simulink model "Project_SADC"  (R2021b)
settings: Solver=ode45  StartTime=0.0  StopTime=T  FixedStep=1e-6  RelTol=1e-12
values from neighbouring files (symbols this model uses):
  A = [A_sc,A_sp]    [Main_SADC_10572571.m]
  Abn0 = Anb0'    [Main_SADC_10572571.m]
  epsilon = deg2rad(23.45)    [Main_SADC_10572571.m]
  m = [0.01 0.05 0.01]'    [Main_SADC_10572571.m]
  N = [n1 n2 n3 n4 n5 n6 n7 n8 n9 n10]    [Main_SADC_10572571.m]
  n_sun = 2*pi / T_sun    (= 1.99238499086e-07)    [Main_SADC_10572571.m]
  P_srp = Fe_tot/c    [Main_SADC_10572571.m]
  R3H0 = data.Re^3*H0    [Main_SADC_10572571.m]
  R_sun = astroConstants(2)    [Main_SADC_10572571.m]
  rho_d = cat(2,ones(1,6)*rho_d_sc,ones(1,4)*rho_d_sp)    [Main_SADC_10572571.m]
  rho_s = cat(2,ones(1,6)*rho_s_sc,ones(1,4)*rho_s_sp)    [Main_SADC_10572571.m]
  ri = [ri_sc,r_sp1,r_sp1,r_sp2,r_sp2]    [Main_SADC_10572571.m]
  w0 = [wx0 wy0 wz0]'    [Main_SADC_10572571.m]
  weights = [0.15;0.5;0.35]    [Main_SADC_10572571.m]
undefined symbols (not defined in the file or in its folder): data, gyro, horizonsensor, magnetometer, rr0, sc, sunsensor, vv0, wheel
libraries: simulink_extras x10
(part 2 of 3)

== system Project_SADC/Attitude determination /selection sensor/If Action Subsystem3 ==
  In1 : Inport
  Action Port : ActionPort
  Out1 : Outport
  wires:
  In1/1 -> Out1/1

== system Project_SADC/Attitude determination /selection sensor/Vector norm3 ==
  u : Inport
  Divide : Product  Inputs=*/
  norm_vector : Subsystem
  u_versor : Outport
  ||u|| : Outport  Port=2
  wires:
  Divide/1 -> u_versor/1
  norm_vector/1(|u|) -> Divide/2, ||u||/1
  u/1 -> norm_vector/1(u), Divide/1

== system Project_SADC/Euler equations/product vector/i-component ==
  A : Inport
  B : Inport  Port=2
  Demux : Demux  Outputs=3
  Demux1 : Demux  Outputs=3
  Product : Product
  Product1 : Product
  Sum : Sum  Inputs=+-
  Terminator : Terminator
  Terminator1 : Terminator
  Out2 : Outport
  wires:
  Sum/1 -> Out2/1
  Product1/1 -> Sum/2  "a3b2"
  Demux1/2 -> Product1/2  "b2"
  Product/1 -> Sum/1  "a2b3"
  Demux/2 -> Product/1  "a2"
  Demux/3 -> Product1/1  "a3"
  Demux1/3 -> Product/2  "b3"
  Demux/1 -> Terminator/1  "a1"
  Demux1/1 -> Terminator1/1
  B/1 -> Demux1/1
  A/1 -> Demux/1

== system Project_SADC/Euler equations/product vector/j-component ==
  A : Inport
  B : Inport  Port=2
  Demux : Demux  Outputs=3
  Demux1 : Demux  Outputs=3
  Product : Product
  Product1 : Product
  Sum : Sum  Inputs=+-
  Terminator : Terminator
  Terminator1 : Terminator
  Out1 : Outport
  wires:
  B/1 -> Demux1/1
  A/1 -> Demux/1
  Demux/3 -> Product/1  "a3"
  Demux1/1 -> Product/2  "b1"
  Demux/1 -> Product1/1  "a1"
  Demux1/3 -> Product1/2  "b3"
  Demux1/2 -> Terminator/1
  Demux/2 -> Terminator1/1
  Product/1 -> Sum/1
  Product1/1 -> Sum/2
  Sum/1 -> Out1/1

== system Project_SADC/Euler equations/product vector/k-component1 ==
  A : Inport
  B : Inport  Port=2
  Demux : Demux  Outputs=3
  Demux1 : Demux  Outputs=3
  Product : Product
  Product1 : Product
  Sum : Sum  Inputs=+-
  Terminator : Terminator
  Terminator1 : Terminator
  Out1 : Outport
  wires:
  Sum/1 -> Out1/1
  Product1/1 -> Sum/2
  Product/1 -> Sum/1
  Demux1/2 -> Product/2  "b2"
  A/1 -> Demux/1
  B/1 -> Demux1/1
  Demux/1 -> Product/1  "a1"
  Demux/2 -> Product1/1  "a2"
  Demux1/1 -> Product1/2  "b1"
  Demux1/3 -> Terminator/1  "b3"
  Demux/3 -> Terminator1/1  "a3"

== system Project_SADC/External torques/GG torque/Vector norm ==
  u : Inport
  Divide : Product  Inputs=*/
  norm_vector : Subsystem
  u_versor : Outport
  ||u|| : Outport  Port=2
  wires:
  u/1 -> Divide/1, norm_vector/1(u)
  norm_vector/1(|u|) -> ||u||/1, Divide/2
  Divide/1 -> u_versor/1

== system Project_SADC/External torques/GG torque/product vector ==
  A : Inport
  B : Inport  Port=2
  Mux : Mux  Inputs=3
  i-component : Subsystem
  j-component : Subsystem
  k-component1 : Subsystem
  C : Outport
  wires:
  Mux/1 -> C/1
  A/1 -> k-component1/1(A), j-component/1(A), i-component/1(A)
  B/1 -> k-component1/2(B), j-component/2(B), i-component/2(B)
  i-component/1(Out2) -> Mux/1
  j-component/1(Out1) -> Mux/2
  k-component1/1(Out1) -> Mux/3

== system Project_SADC/External torques/Magnetic torque/mag_field in inertial ==
  r_vect : Inport
  time : Inport  Port=2
  Constant : Constant  Value=3
  Constant1 : Constant  Value=R3H0
  Dot Product : DotProduct  InputSameDT=on  OutDataTypeStr=Inherit: Inherit via internal rule
  Gain : Gain  Gain=3
  MatrixMultiply : Product
  MatrixMultiply1 : Product
  Power : Math  Operator=pow  SaturateOnIntegerOverflow=on
  Product : Product  Inputs=/*
  Sum : Sum  Inputs=+-
  Vector norm1 : Subsystem
  m_versor : Subsystem
  b_B : Outport
  wires:
  r_vect/1 -> Vector norm1/1(u)
  time/1 -> m_versor/1(time)
  Vector norm1/2(||u||) -> Power/1
  Constant/1 -> Power/2
  Power/1 -> Product/1
  Constant1/1 -> Product/2
  m_versor/1(m) -> Sum/2, Dot Product/1
  Vector norm1/1(u_versor) -> MatrixMultiply/2, Dot Product/2
  MatrixMultiply/1 -> Sum/1
  Sum/1 -> MatrixMultiply1/1
  Product/1 -> MatrixMultiply1/2
  MatrixMultiply1/1 -> b_B/1
  Dot Product/1 -> Gain/1
  Gain/1 -> MatrixMultiply/1

== system Project_SADC/External torques/Magnetic torque/product vector2 ==
  A : Inport
  B : Inport  Port=2
  Mux : Mux  Inputs=3
  i-component : Subsystem
  j-component : Subsystem
  k-component1 : Subsystem
  C : Outport
  wires:
  k-component1/1(Out1) -> Mux/3
  j-component/1(Out1) -> Mux/2
  i-component/1(Out2) -> Mux/1
  B/1 -> i-component/2(B), j-component/2(B), k-component1/2(B)
  A/1 -> i-component/1(A), j-component/1(A), k-component1/1(A)
  Mux/1 -> C/1

== system Project_SADC/External torques/SRP torque/SRP forces ==
  r_Sun : Inport
  Constant : Constant  Value=1-rho_s  VectorParams1D=off
  Constant1 : Constant  Value=2.*rho_s  VectorParams1D=off
  Constant2 : Constant  Value=N  VectorParams1D=off
  Constant3 : Constant  Value=rho_d.*2./3  VectorParams1D=off
  Constant4 : Constant  Value=ones(1,10)  VectorParams1D=off
  Constant5 : Constant  Value=A  VectorParams1D=off
  Display : Display
  Element-wise([1x9].*[3x9])1 : Subsystem
  Element-wise([1x9].*[3x9])2 : Subsystem
  Element-wise([1x9].*[3x9])3 : Subsystem
  Gain : Gain  Gain=-P_srp
  MatrixMultiply : Product
  MatrixMultiply1 : Product  Multiplication=Matrix(*)
  MatrixMultiply2 : Product
  Subsystem : Subsystem
  Sum : Sum
  Sum1 : Sum
  Terminator : Terminator
  Vector norm1 : Subsystem
  F_srp : Outport
  S_dot_N : Outport  Port=2
  wires:
  Subsystem/1(S_dot_N) -> MatrixMultiply2/1, S_dot_N/1, MatrixMultiply/2
  Constant1/1 -> MatrixMultiply/1
  MatrixMultiply/1 -> Sum/2
  Constant3/1 -> Sum/1
  Constant2/1 -> Element-wise([1x9].*[3x9])3/1(N), Subsystem/2(N)
  Sum/1 -> Element-wise([1x9].*[3x9])3/2(vector)
  Constant4/1 -> MatrixMultiply1/2
  MatrixMultiply1/1 -> Element-wise([1x9].*[3x9])1/1(Sb)
  Constant/1 -> Display/1, Element-wise([1x9].*[3x9])1/2(vector)
  Element-wise([1x9].*[3x9])1/1(vect.*Sb) -> Sum1/1
  Element-wise([1x9].*[3x9])3/1(vect.*n) -> Sum1/2
  Constant5/1 -> Gain/1
  Gain/1 -> MatrixMultiply2/2
  Sum1/1 -> Element-wise([1x9].*[3x9])2/1(mat)
  MatrixMultiply2/1 -> Element-wise([1x9].*[3x9])2/2(vector)
  Element-wise([1x9].*[3x9])2/1(vect.*mat) -> F_srp/1
  r_Sun/1 -> Vector norm1/1(u)
  Vector norm1/1(u_versor) -> MatrixMultiply1/1, Subsystem/1(r_sun)
  Vector norm1/2(||u||) -> Terminator/1

== system Project_SADC/External torques/SRP torque/Sun wrt s//c ==
  A_BN : Inport
  r_vect : Inport  Port=2
  t : Inport  Port=3
  MatrixMultiply : Product  Multiplication=Matrix(*)
  R_Sun in inertial : Subsystem
  Sum : Sum  Inputs=-+
  To Workspace : ToWorkspace  VariableName=r_Sun_N  SaveFormat=Timeseries  SampleTime=-1
  r_sun : Outport
  rSun_N : Outport  Port=2
  wires:
  t/1 -> R_Sun in inertial/1(t)
  r_vect/1 -> Sum/1
  R_Sun in inertial/1(R_sun_N) -> rSun_N/1, To Workspace/1, Sum/2
  Sum/1 -> MatrixMultiply/2
  A_BN/1 -> MatrixMultiply/1
  MatrixMultiply/1 -> r_sun/1  "R_Sun in body"

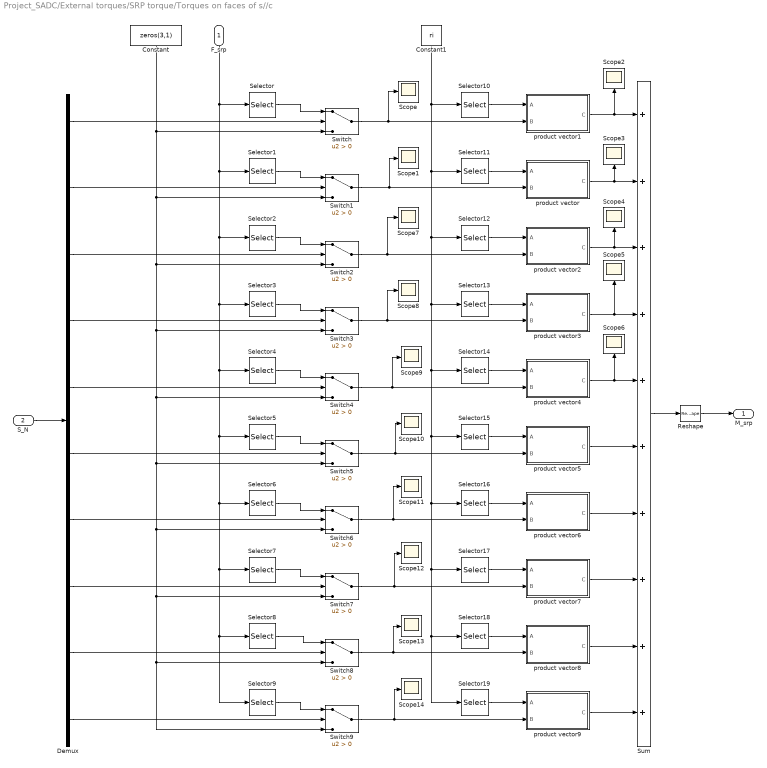
== system Project_SADC/External torques/SRP torque/Torques on faces of s//c ==
  F_srp : Inport
  S_N : Inport  Port=2
  Constant : Constant  Value=zeros(3,1)
  Constant1 : Constant  Value=ri
  Demux : Demux  Outputs=10
  Reshape : Reshape  OutputDimensionality=Column vector (2-D)
  Scope{,1..14} (15 alike) : Scope
  Selector : Selector  NumberOfDimensions=2  InputPortWidth=3  IndexOptions=Index vector (dialog),Index vector (dialog)  Indices=[1 2 3],1  OutputSizes=1,1
  Selector1 : Selector  NumberOfDimensions=2  InputPortWidth=3  IndexOptions=Index vector (dialog),Index vector (dialog)  Indices=[1 2 3],2  OutputSizes=1,1
  Selector10 : Selector  NumberOfDimensions=2  InputPortWidth=3  IndexOptions=Index vector (dialog),Index vector (dialog)  Indices=[1 2 3],1  OutputSizes=1,1
  Selector11 : Selector  NumberOfDimensions=2  InputPortWidth=3  IndexOptions=Index vector (dialog),Index vector (dialog)  Indices=[1 2 3],2  OutputSizes=1,1
  Selector12 : Selector  NumberOfDimensions=2  InputPortWidth=3  IndexOptions=Index vector (dialog),Index vector (dialog)  Indices=[1 2 3],3  OutputSizes=1,1
  Selector13 : Selector  NumberOfDimensions=2  InputPortWidth=3  IndexOptions=Index vector (dialog),Index vector (dialog)  Indices=[1 2 3],4  OutputSizes=1,1
  Selector14 : Selector  NumberOfDimensions=2  InputPortWidth=3  IndexOptions=Index vector (dialog),Index vector (dialog)  Indices=[1 2 3],5  OutputSizes=1,1
  Selector15 : Selector  NumberOfDimensions=2  InputPortWidth=3  IndexOptions=Index vector (dialog),Index vector (dialog)  Indices=[1 2 3],6  OutputSizes=1,1
  Selector16 : Selector  NumberOfDimensions=2  InputPortWidth=3  IndexOptions=Index vector (dialog),Index vector (dialog)  Indices=[1 2 3],7  OutputSizes=1,1
  Selector17 : Selector  NumberOfDimensions=2  InputPortWidth=3  IndexOptions=Index vector (dialog),Index vector (dialog)  Indices=[1 2 3],8  OutputSizes=1,1
  Selector18 : Selector  NumberOfDimensions=2  InputPortWidth=3  IndexOptions=Index vector (dialog),Index vector (dialog)  Indices=[1 2 3],9  OutputSizes=1,1
  Selector19 : Selector  NumberOfDimensions=2  InputPortWidth=3  IndexOptions=Index vector (dialog),Index vector (dialog)  Indices=[1 2 3],10  OutputSizes=1,1
  Selector2 : Selector  NumberOfDimensions=2  InputPortWidth=3  IndexOptions=Index vector (dialog),Index vector (dialog)  Indices=[1 2 3],3  OutputSizes=1,1
  Selector3 : Selector  NumberOfDimensions=2  InputPortWidth=3  IndexOptions=Index vector (dialog),Index vector (dialog)  Indices=[1 2 3],4  OutputSizes=1,1
  Selector4 : Selector  NumberOfDimensions=2  InputPortWidth=3  IndexOptions=Index vector (dialog),Index vector (dialog)  Indices=[1 2 3],5  OutputSizes=1,1
  Selector5 : Selector  NumberOfDimensions=2  InputPortWidth=3  IndexOptions=Index vector (dialog),Index vector (dialog)  Indices=[1 2 3],6  OutputSizes=1,1
  Selector6 : Selector  NumberOfDimensions=2  InputPortWidth=3  IndexOptions=Index vector (dialog),Index vector (dialog)  Indices=[1 2 3],7  OutputSizes=1,1
  Selector7 : Selector  NumberOfDimensions=2  InputPortWidth=3  IndexOptions=Index vector (dialog),Index vector (dialog)  Indices=[1 2 3],8  OutputSizes=1,1
  Selector8 : Selector  NumberOfDimensions=2  InputPortWidth=3  IndexOptions=Index vector (dialog),Index vector (dialog)  Indices=[1 2 3],9  OutputSizes=1,1
  Selector9 : Selector  NumberOfDimensions=2  InputPortWidth=3  IndexOptions=Index vector (dialog),Index vector (dialog)  Indices=[1 2 3],10  OutputSizes=1,1
  Sum : Sum  Inputs=++++++++++
  Switch{,1..9} (10 alike) : Switch  Criteria=u2 > Threshold
  product vector : Subsystem
  product vector1 : Subsystem
  product vector2 : Subsystem
  product vector3 : Subsystem
  product vector4 : Subsystem
  product vector5 : Subsystem
  product vector6 : Subsystem
  product vector7 : Subsystem
  product vector8 : Subsystem
  product vector9 : Subsystem
  M_srp : Outport
  wires:
  S_N/1 -> Demux/1
  Demux/1 -> Switch/2
  F_srp/1 -> Selector9/1, Selector8/1, Selector7/1, Selector6/1, Selector5/1, Selector4/1, Selector3/1, Selector2/1, Selector1/1, Selector/1
  Selector/1 -> Switch/1
  Constant/1 -> Switch4/3, Switch9/3, Switch8/3, Switch7/3, Switch6/3, Switch5/3, Switch3/3, Switch2/3, Switch1/3, Switch/3
  Demux/2 -> Switch1/2
  Selector1/1 -> Switch1/1
  Demux/3 -> Switch2/2
  Selector2/1 -> Switch2/1
  Demux/4 -> Switch3/2
  Demux/5 -> Switch4/2
  Selector3/1 -> Switch3/1
  Selector4/1 -> Switch4/1
  Demux/6 -> Switch5/2
  Selector5/1 -> Switch5/1
  Demux/7 -> Switch6/2
  Selector6/1 -> Switch6/1
  Demux/8 -> Switch7/2
  Selector7/1 -> Switch7/1
  Demux/9 -> Switch8/2
  Selector8/1 -> Switch8/1
  Demux/10 -> Switch9/2
  Selector9/1 -> Switch9/1
  Selector10/1 -> product vector1/1(A)
  Switch/1 -> Scope/1, product vector1/2(B)
  Selector11/1 -> product vector/1(A)
  Switch1/1 -> Scope1/1, product vector/2(B)
  Selector12/1 -> product vector2/1(A)
  Switch3/1 -> Scope8/1, product vector3/2(B)
  Selector13/1 -> product vector3/1(A)
  Switch4/1 -> Scope9/1, product vector4/2(B)
  Selector14/1 -> product vector4/1(A)
  Switch5/1 -> Scope10/1, product vector5/2(B)
  Selector15/1 -> product vector5/1(A)
  Switch6/1 -> Scope11/1, product vector6/2(B)
  Selector16/1 -> product vector6/1(A)
  Switch7/1 -> Scope12/1, product vector7/2(B)
  Selector17/1 -> product vector7/1(A)
  Switch8/1 -> Scope13/1, product vector8/2(B)
  Selector18/1 -> product vector8/1(A)
  Switch9/1 -> Scope14/1, product vector9/2(B)
  Selector19/1 -> product vector9/1(A)
  Constant1/1 -> Selector19/1, Selector18/1, Selector17/1, Selector16/1, Selector15/1, Selector14/1, Selector13/1, Selector12/1, Selector11/1, Selector10/1
  product vector9/1(C) -> Sum/10
  product vector1/1(C) -> Sum/1, Scope2/1
  product vector/1(C) -> Scope3/1, Sum/2
  product vector2/1(C) -> Scope4/1, Sum/3
  product vector3/1(C) -> Scope5/1, Sum/4
  product vector7/1(C) -> Sum/8
  product vector6/1(C) -> Sum/7
  product vector5/1(C) -> Sum/6
  product vector4/1(C) -> Scope6/1, Sum/5
  product vector8/1(C) -> Sum/9
  Sum/1 -> Reshape/1
  Reshape/1 -> M_srp/1
  Switch2/1 -> Scope7/1, product vector2/2(B)

== system Project_SADC/External torques/Vector norm/norm_vector ==
  u : Inport
  Demux : Demux  Outputs=3
  Square : Math  Operator=square  SaturateOnIntegerOverflow=on
  Square Root : Sqrt  SaturateOnIntegerOverflow=on
  Square1 : Math  Operator=square  SaturateOnIntegerOverflow=on
  Square3 : Math  Operator=square  SaturateOnIntegerOverflow=on
  Sum : Sum  Inputs=+++
  |u| : Outport
  wires:
  u/1 -> Demux/1
  Demux/1 -> Square/1
  Demux/2 -> Square1/1
  Demux/3 -> Square3/1
  Square/1 -> Sum/1
  Square3/1 -> Sum/3
  Square1/1 -> Sum/2
  Sum/1 -> Square Root/1
  Square Root/1 -> |u|/1

== system Project_SADC/Orbit/Orbit integration /Subsystem1 ==
  u : Inport
  Divide : Product  Inputs=*/
  norm_vector : Subsystem
  u_versor : Outport
  ||u|| : Outport  Port=2
  wires:
  u/1 -> Divide/1, norm_vector/1(u)
  norm_vector/1(|u|) -> ||u||/1, Divide/2
  Divide/1 -> u_versor/1

== system Project_SADC/Orbit/product vector/i-component ==
  A : Inport
  B : Inport  Port=2
  Demux : Demux  Outputs=3
  Demux1 : Demux  Outputs=3
  Product : Product
  Product1 : Product
  Sum : Sum  Inputs=+-
  Terminator : Terminator
  Terminator1 : Terminator
  Out2 : Outport
  wires:
  Sum/1 -> Out2/1
  Product1/1 -> Sum/2  "a3b2"
  Demux1/2 -> Product1/2  "b2"
  Product/1 -> Sum/1  "a2b3"
  Demux/2 -> Product/1  "a2"
  Demux/3 -> Product1/1  "a3"
  Demux1/3 -> Product/2  "b3"
  Demux/1 -> Terminator/1  "a1"
  Demux1/1 -> Terminator1/1
  B/1 -> Demux1/1
  A/1 -> Demux/1

== system Project_SADC/Orbit/product vector/j-component ==
  A : Inport
  B : Inport  Port=2
  Demux : Demux  Outputs=3
  Demux1 : Demux  Outputs=3
  Product : Product
  Product1 : Product
  Sum : Sum  Inputs=+-
  Terminator : Terminator
  Terminator1 : Terminator
  Out1 : Outport
  wires:
  B/1 -> Demux1/1
  A/1 -> Demux/1
  Demux/3 -> Product/1  "a3"
  Demux1/1 -> Product/2  "b1"
  Demux/1 -> Product1/1  "a1"
  Demux1/3 -> Product1/2  "b3"
  Demux1/2 -> Terminator/1
  Demux/2 -> Terminator1/1
  Product/1 -> Sum/1
  Product1/1 -> Sum/2
  Sum/1 -> Out1/1

== system Project_SADC/Orbit/product vector/k-component1 ==
  A : Inport
  B : Inport  Port=2
  Demux : Demux  Outputs=3
  Demux1 : Demux  Outputs=3
  Product : Product
  Product1 : Product
  Sum : Sum  Inputs=+-
  Terminator : Terminator
  Terminator1 : Terminator
  Out1 : Outport
  wires:
  Sum/1 -> Out1/1
  Product1/1 -> Sum/2
  Product/1 -> Sum/1
  Demux1/2 -> Product/2  "b2"
  A/1 -> Demux/1
  B/1 -> Demux1/1
  Demux/1 -> Product/1  "a1"
  Demux/2 -> Product1/1  "a2"
  Demux1/1 -> Product1/2  "b1"
  Demux1/3 -> Terminator/1  "b3"
  Demux/3 -> Terminator1/1  "a3"

== system Project_SADC/Reaction Wheels/product vector1/i-component ==
  A : Inport
  B : Inport  Port=2
  Demux : Demux  Outputs=3
  Demux1 : Demux  Outputs=3
  Product : Product
  Product1 : Product
  Sum : Sum  Inputs=+-
  Terminator : Terminator
  Terminator1 : Terminator
  Out2 : Outport
  wires:
  A/1 -> Demux/1
  B/1 -> Demux1/1
  Demux1/1 -> Terminator1/1
  Demux/1 -> Terminator/1  "a1"
  Demux1/3 -> Product/2  "b3"
  Demux/3 -> Product1/1  "a3"
  Demux/2 -> Product/1  "a2"
  Product/1 -> Sum/1  "a2b3"
  Demux1/2 -> Product1/2  "b2"
  Product1/1 -> Sum/2  "a3b2"
  Sum/1 -> Out2/1

== system Project_SADC/Reaction Wheels/product vector1/j-component ==
  A : Inport
  B : Inport  Port=2
  Demux : Demux  Outputs=3
  Demux1 : Demux  Outputs=3
  Product : Product
  Product1 : Product
  Sum : Sum  Inputs=+-
  Terminator : Terminator
  Terminator1 : Terminator
  Out1 : Outport
  wires:
  Sum/1 -> Out1/1
  Product1/1 -> Sum/2
  Product/1 -> Sum/1
  Demux/2 -> Terminator1/1
  Demux1/2 -> Terminator/1
  Demux1/3 -> Product1/2  "b3"
  Demux/1 -> Product1/1  "a1"
  Demux1/1 -> Product/2  "b1"
  Demux/3 -> Product/1  "a3"
  A/1 -> Demux/1
  B/1 -> Demux1/1

== system Project_SADC/Reaction Wheels/product vector1/k-component1 ==
  A : Inport
  B : Inport  Port=2
  Demux : Demux  Outputs=3
  Demux1 : Demux  Outputs=3
  Product : Product
  Product1 : Product
  Sum : Sum  Inputs=+-
  Terminator : Terminator
  Terminator1 : Terminator
  Out1 : Outport
  wires:
  Demux/3 -> Terminator1/1  "a3"
  Demux1/3 -> Terminator/1  "b3"
  Demux1/1 -> Product1/2  "b1"
  Demux/2 -> Product1/1  "a2"
  Demux/1 -> Product/1  "a1"
  B/1 -> Demux1/1
  A/1 -> Demux/1
  Demux1/2 -> Product/2  "b2"
  Product/1 -> Sum/1
  Product1/1 -> Sum/2
  Sum/1 -> Out1/1

== system Project_SADC/Reaction Wheels/product vector4/i-component ==
  A : Inport
  B : Inport  Port=2
  Demux : Demux  Outputs=3
  Demux1 : Demux  Outputs=3
  Product : Product
  Product1 : Product
  Sum : Sum  Inputs=+-
  Terminator : Terminator
  Terminator1 : Terminator
  Out2 : Outport
  wires:
  Sum/1 -> Out2/1
  Product1/1 -> Sum/2  "a3b2"
  Demux1/2 -> Product1/2  "b2"
  Product/1 -> Sum/1  "a2b3"
  Demux/2 -> Product/1  "a2"
  Demux/3 -> Product1/1  "a3"
  Demux1/3 -> Product/2  "b3"
  Demux/1 -> Terminator/1  "a1"
  Demux1/1 -> Terminator1/1
  B/1 -> Demux1/1
  A/1 -> Demux/1

== system Project_SADC/Reaction Wheels/product vector4/j-component ==
  A : Inport
  B : Inport  Port=2
  Demux : Demux  Outputs=3
  Demux1 : Demux  Outputs=3
  Product : Product
  Product1 : Product
  Sum : Sum  Inputs=+-
  Terminator : Terminator
  Terminator1 : Terminator
  Out1 : Outport
  wires:
  B/1 -> Demux1/1
  A/1 -> Demux/1
  Demux/3 -> Product/1  "a3"
  Demux1/1 -> Product/2  "b1"
  Demux/1 -> Product1/1  "a1"
  Demux1/3 -> Product1/2  "b3"
  Demux1/2 -> Terminator/1
  Demux/2 -> Terminator1/1
  Product/1 -> Sum/1
  Product1/1 -> Sum/2
  Sum/1 -> Out1/1

== system Project_SADC/Reaction Wheels/product vector4/k-component1 ==
  A : Inport
  B : Inport  Port=2
  Demux : Demux  Outputs=3
  Demux1 : Demux  Outputs=3
  Product : Product
  Product1 : Product
  Sum : Sum  Inputs=+-
  Terminator : Terminator
  Terminator1 : Terminator
  Out1 : Outport
  wires:
  Sum/1 -> Out1/1
  Product1/1 -> Sum/2
  Product/1 -> Sum/1
  Demux1/2 -> Product/2  "b2"
  A/1 -> Demux/1
  B/1 -> Demux1/1
  Demux/1 -> Product/1  "a1"
  Demux/2 -> Product1/1  "a2"
  Demux1/1 -> Product1/2  "b1"
  Demux1/3 -> Terminator/1  "b3"
  Demux/3 -> Terminator1/1  "a3"

== system Project_SADC/Relative Attitude/DCM from L to B and from L to N/DCM from L to N ==
  r_vect : Inport
  h_vect : Inport  Port=2
  Display{,1..3} (4 alike) : Display
  Gain : Gain  Gain=-1
  Mux : Mux  Inputs=3
  Reshape : Reshape  OutputDimensionality=Customize  OutputDimensions=[3,3]
  Terminator : Terminator
  Terminator1 : Terminator
  Vector norm : Subsystem
  Vector norm1 : Subsystem
  product vector : Subsystem
  A_NL : Outport
  wires:
  r_vect/1 -> Vector norm/1(u)
  h_vect/1 -> Vector norm1/1(u)
  Vector norm/2(||u||) -> Terminator/1
  Vector norm1/2(||u||) -> Terminator1/1
  Vector norm/1(u_versor) -> Mux/1, Display/1, product vector/1(A)
  Vector norm1/1(u_versor) -> Mux/3, Display3/1, product vector/2(B)
  Mux/1 -> Reshape/1
  product vector/1(C) -> Gain/1
  Gain/1 -> Mux/2, Display2/1
  Reshape/1 -> A_NL/1, Display1/1

== system Project_SADC/Relative Attitude/DCM from L to B and from L to N/Vector norm ==
  u : Inport
  Divide : Product  Inputs=*/
  norm_vector : Subsystem
  u_versor : Outport
  ||u|| : Outport  Port=2
  wires:
  u/1 -> Divide/1, norm_vector/1(u)
  norm_vector/1(|u|) -> ||u||/1, Divide/2
  Divide/1 -> u_versor/1

== system Project_SADC/Relative Attitude/DCM from L to B and from L to N/Vector norm1 ==
  u : Inport
  Divide : Product  Inputs=*/
  norm_vector : Subsystem
  u_versor : Outport
  ||u|| : Outport  Port=2
  wires:
  Divide/1 -> u_versor/1
  norm_vector/1(|u|) -> Divide/2, ||u||/1
  u/1 -> norm_vector/1(u), Divide/1

== system Project_SADC/Sensors/Check if in EH FOV/If Action Subsystem ==
  u_versor : Inport
  Action Port : ActionPort  ActionPortLabel=if(u1 > 90)
  Gain : Gain  Gain=0
  Out1 : Outport
  wires:
  Gain/1 -> Out1/1
  u_versor/1 -> Gain/1

== system Project_SADC/Sensors/Check if in EH FOV/If Action Subsystem1 ==
  u_versor : Inport
  Action Port : ActionPort  ActionPortLabel=else
  Out1 : Outport
  wires:
  u_versor/1 -> Out1/1

== system Project_SADC/Sensors/Check if in EH FOV/Vector norm1 ==
  u : Inport
  Divide : Product  Inputs=*/
  norm_vector : Subsystem
  u_versor : Outport
  ||u|| : Outport  Port=2
  wires:
  u/1 -> Divide/1, norm_vector/1(u)
  norm_vector/1(|u|) -> ||u||/1, Divide/2
  Divide/1 -> u_versor/1

== system Project_SADC/Sensors/Check if in sunsensor FOV/If Action Subsystem ==
  In1 : Inport
  Action Port : ActionPort  ActionPortLabel=if(u1 > 60)
  Gain : Gain  Gain=0
  Out1 : Outport
  wires:
  In1/1 -> Gain/1
  Gain/1 -> Out1/1

== system Project_SADC/Sensors/Check if in sunsensor FOV/If Action Subsystem1 ==
  In1 : Inport
  Action Port : ActionPort  ActionPortLabel=else
  Out1 : Outport
  wires:
  In1/1 -> Out1/1

== system Project_SADC/Sensors/Check if in sunsensor FOV/Vector norm1 ==
  u : Inport
  Divide : Product  Inputs=*/
  norm_vector : Subsystem
  u_versor : Outport
  ||u|| : Outport  Port=2
  wires:
  Divide/1 -> u_versor/1
  norm_vector/1(|u|) -> Divide/2, ||u||/1
  u/1 -> norm_vector/1(u), Divide/1

== system Project_SADC/Sensors/Cylindrical eclipse model/If Action Subsystem ==
  In1 : Inport
  Action Port : ActionPort
  Out1 : Outport
  wires:
  In1/1 -> Out1/1

== system Project_SADC/Sensors/Cylindrical eclipse model/If Action Subsystem1 ==
  u_versor : Inport
  Action Port : ActionPort
  Output1 : Outport
  wires:
  u_versor/1 -> Output1/1

== system Project_SADC/Sensors/Cylindrical eclipse model/Vec tor norm2 ==
  u : Inport
  Divide : Product  Inputs=*/
  norm_vector : Subsystem
  u_versor : Outport
  ||u|| : Outport  Port=2
  wires:
  u/1 -> Divide/1, norm_vector/1(u)
  norm_vector/1(|u|) -> ||u||/1, Divide/2
  Divide/1 -> u_versor/1

== system Project_SADC/Sensors/Cylindrical eclipse model/Vector norm1 ==
  u : Inport
  Divide : Product  Inputs=*/
  norm_vector : Subsystem
  u_versor : Outport
  ||u|| : Outport  Port=2
  wires:
  Divide/1 -> u_versor/1
  norm_vector/1(|u|) -> Divide/2, ||u||/1
  u/1 -> norm_vector/1(u), Divide/1

== system Project_SADC/Sensors/Cylindrical eclipse model/Vector norm2 ==
  u : Inport
  Divide : Product  Inputs=*/
  norm_vector : Subsystem
  u_versor : Outport
  ||u|| : Outport  Port=2
  wires:
  u/1 -> Divide/1, norm_vector/1(u)
  norm_vector/1(|u|) -> ||u||/1, Divide/2
  Divide/1 -> u_versor/1

== system Project_SADC/Sensors/Cylindrical eclipse model/Vector norm3 ==
  u : Inport
  Divide : Product  Inputs=*/
  norm_vector : Subsystem
  u_versor : Outport
  ||u|| : Outport  Port=2
  wires:
  Divide/1 -> u_versor/1
  norm_vector/1(|u|) -> Divide/2, ||u||/1
  u/1 -> norm_vector/1(u), Divide/1

== system Project_SADC/Sensors/Earth horizon/A_eps ==
  Constant : Constant
  Degrees to Radians : simulink_extras/Transformations/Degrees to Radians
  Degrees to Radians1 : simulink_extras/Transformations/Degrees to Radians
  Degrees to Radians2 : simulink_extras/Transformations/Degrees to Radians
  Display : Display
  Gain1 : Gain  Gain=-1
  Gain3 : Gain  Gain=1/10
  Gain4 : Gain  Gain=1/10
  Gain5 : Gain  Gain=1/10
  Gain6 : Gain  Gain=-1
  Gain7 : Gain  Gain=-1
  Mux : Mux  Inputs=9
  Random Number : RandomNumber  Variance=horizonsensor.accuracy^2  Seed=randi([0 400],1,1)  SampleTime=horizonsensor.samplingtime
  Random Number1 : RandomNumber  Variance=horizonsensor.accuracy^2  Seed=randi([0 400],1,1)  SampleTime=horizonsensor.samplingtime
  Random Number2 : RandomNumber  Variance=horizonsensor.accuracy^2  Seed=randi([0 400],1,1)  SampleTime=horizonsensor.samplingtime
  Reshape : Reshape  OutputDimensionality=Customize  OutputDimensions=[3,3]
  Out1 : Outport
  wires:
  Mux/1 -> Reshape/1
  Reshape/1 -> Out1/1, Display/1
  Constant/1 -> Mux/1, Mux/5, Mux/9
  Gain5/1 -> Degrees to Radians2/1
  Gain3/1 -> Degrees to Radians/1
  Gain4/1 -> Degrees to Radians1/1
  Random Number/1 -> Gain3/1
  Random Number1/1 -> Gain4/1
  Random Number2/1 -> Gain5/1
  Gain6/1 -> Mux/3
  Gain7/1 -> Mux/4
  Gain1/1 -> Mux/8
  Degrees to Radians/1 -> Mux/6, Gain1/1
  Degrees to Radians1/1 -> Mux/7, Gain6/1
  Degrees to Radians2/1 -> Mux/2, Gain7/1

== system Project_SADC/Sensors/Gyroscope/Gyroscope1 ==
  w_b : Inport
  Integrator : Integrator
  Random Number : RandomNumber  Variance=(gyro.ARW/sqrt(3600)*pi/180*sqrt(gyro.samplingtime))^2  SampleTime=gyro.samplingtime  VectorParams1D=off
  Random Number1 : RandomNumber  Variance=(gyro.bias/3600*pi/180*sqrt(gyro.samplingtime))^2  SampleTime=gyro.samplingtime
  Sum : Sum  Inputs=+|+|+
  Zero-Order Hold : ZeroOrderHold  SampleTime=1/20
  w_sens : Outport
  wires:
  w_b/1 -> Sum/1
  Sum/1 -> Zero-Order Hold/1
  Random Number/1 -> Sum/2
  Zero-Order Hold/1 -> w_sens/1
  Integrator/1 -> Sum/3
  Random Number1/1 -> Integrator/1

== system Project_SADC/Sensors/Sun sensor/A_eps ==
  Constant : Constant
  Degrees to Radians : simulink_extras/Transformations/Degrees to Radians
  Degrees to Radians1 : simulink_extras/Transformations/Degrees to Radians
  Degrees to Radians2 : simulink_extras/Transformations/Degrees to Radians
  Display : Display
  Gain1 : Gain  Gain=-1
  Gain3 : Gain
  Gain4 : Gain
  Gain5 : Gain
  Gain6 : Gain  Gain=-1
  Gain7 : Gain  Gain=-1
  Mux : Mux  Inputs=9
  Random Number : RandomNumber  Variance=(sunsensor.accuracy)^2  Seed=randi([0 400],1,1)  SampleTime=sunsensor.samplingtime
  Random Number1 : RandomNumber  Variance=(sunsensor.accuracy)^2  Seed=randi([0 400],1,1)  SampleTime=sunsensor.samplingtime
  Random Number2 : RandomNumber  Variance=(sunsensor.accuracy)^2  Seed=randi([0 400],1,1)  SampleTime=sunsensor.samplingtime
  Reshape : Reshape  OutputDimensionality=Customize  OutputDimensions=[3,3]
  Scope : Scope
  Out1 : Outport
  wires:
  Mux/1 -> Reshape/1
  Reshape/1 -> Out1/1, Display/1
  Constant/1 -> Mux/1, Mux/5, Mux/9
  Gain5/1 -> Degrees to Radians2/1
  Gain3/1 -> Degrees to Radians/1
  Gain4/1 -> Degrees to Radians1/1
  Random Number/1 -> Scope/1, Gain3/1
  Random Number1/1 -> Gain4/1
  Random Number2/1 -> Gain5/1
  Gain6/1 -> Mux/3
  Gain7/1 -> Mux/4
  Gain1/1 -> Mux/8
  Degrees to Radians/1 -> Mux/6, Gain1/1
  Degrees to Radians1/1 -> Mux/7, Gain6/1
  Degrees to Radians2/1 -> Mux/2, Gain7/1

== system Project_SADC/Attitude determination /TRIAD /Vector norm1/norm_vector ==
  u : Inport
  Demux : Demux  Outputs=3
  Square : Math  Operator=square  SaturateOnIntegerOverflow=on
  Square Root : Sqrt  SaturateOnIntegerOverflow=on
  Square1 : Math  Operator=square  SaturateOnIntegerOverflow=on
  Square3 : Math  Operator=square  SaturateOnIntegerOverflow=on
  Sum : Sum  Inputs=+++
  |u| : Outport
  wires:
  u/1 -> Demux/1
  Demux/1 -> Square/1
  Demux/2 -> Square1/1
  Demux/3 -> Square3/1
  Square/1 -> Sum/1
  Square3/1 -> Sum/3
  Square1/1 -> Sum/2
  Sum/1 -> Square Root/1
  Square Root/1 -> |u|/1

== system Project_SADC/Attitude determination /TRIAD /Vector norm2/norm_vector ==
  u : Inport
  Demux : Demux  Outputs=3
  Square : Math  Operator=square  SaturateOnIntegerOverflow=on
  Square Root : Sqrt  SaturateOnIntegerOverflow=on
  Square1 : Math  Operator=square  SaturateOnIntegerOverflow=on
  Square3 : Math  Operator=square  SaturateOnIntegerOverflow=on
  Sum : Sum  Inputs=+++
  |u| : Outport
  wires:
  u/1 -> Demux/1
  Demux/1 -> Square/1
  Demux/2 -> Square1/1
  Demux/3 -> Square3/1
  Square/1 -> Sum/1
  Square3/1 -> Sum/3
  Square1/1 -> Sum/2
  Sum/1 -> Square Root/1
  Square Root/1 -> |u|/1

== system Project_SADC/Attitude determination /TRIAD /product vector2/i-component ==
  A : Inport
  B : Inport  Port=2
  Demux : Demux  Outputs=3
  Demux1 : Demux  Outputs=3
  Product : Product
  Product1 : Product
  Sum : Sum  Inputs=+-
  Terminator : Terminator
  Terminator1 : Terminator
  Out2 : Outport
  wires:
  A/1 -> Demux/1
  B/1 -> Demux1/1
  Demux1/1 -> Terminator1/1
  Demux/1 -> Terminator/1  "a1"
  Demux1/3 -> Product/2  "b3"
  Demux/3 -> Product1/1  "a3"
  Demux/2 -> Product/1  "a2"
  Product/1 -> Sum/1  "a2b3"
  Demux1/2 -> Product1/2  "b2"
  Product1/1 -> Sum/2  "a3b2"
  Sum/1 -> Out2/1

== system Project_SADC/Attitude determination /TRIAD /product vector2/j-component ==
  A : Inport
  B : Inport  Port=2
  Demux : Demux  Outputs=3
  Demux1 : Demux  Outputs=3
  Product : Product
  Product1 : Product
  Sum : Sum  Inputs=+-
  Terminator : Terminator
  Terminator1 : Terminator
  Out1 : Outport
  wires:
  Sum/1 -> Out1/1
  Product1/1 -> Sum/2
  Product/1 -> Sum/1
  Demux/2 -> Terminator1/1
  Demux1/2 -> Terminator/1
  Demux1/3 -> Product1/2  "b3"
  Demux/1 -> Product1/1  "a1"
  Demux1/1 -> Product/2  "b1"
  Demux/3 -> Product/1  "a3"
  A/1 -> Demux/1
  B/1 -> Demux1/1

== system Project_SADC/Attitude determination /TRIAD /product vector2/k-component1 ==
  A : Inport
  B : Inport  Port=2
  Demux : Demux  Outputs=3
  Demux1 : Demux  Outputs=3
  Product : Product
  Product1 : Product
  Sum : Sum  Inputs=+-
  Terminator : Terminator
  Terminator1 : Terminator
  Out1 : Outport
  wires:
  Demux/3 -> Terminator1/1  "a3"
  Demux1/3 -> Terminator/1  "b3"
  Demux1/1 -> Product1/2  "b1"
  Demux/2 -> Product1/1  "a2"
  Demux/1 -> Product/1  "a1"
  B/1 -> Demux1/1
  A/1 -> Demux/1
  Demux1/2 -> Product/2  "b2"
  Product/1 -> Sum/1
  Product1/1 -> Sum/2
  Sum/1 -> Out1/1

== system Project_SADC/Attitude determination /TRIAD /product vector3/i-component ==
  A : Inport
  B : Inport  Port=2
  Demux : Demux  Outputs=3
  Demux1 : Demux  Outputs=3
  Product : Product
  Product1 : Product
  Sum : Sum  Inputs=+-
  Terminator : Terminator
  Terminator1 : Terminator
  Out2 : Outport
  wires:
  Sum/1 -> Out2/1
  Product1/1 -> Sum/2  "a3b2"
  Demux1/2 -> Product1/2  "b2"
  Product/1 -> Sum/1  "a2b3"
  Demux/2 -> Product/1  "a2"
  Demux/3 -> Product1/1  "a3"
  Demux1/3 -> Product/2  "b3"
  Demux/1 -> Terminator/1  "a1"
  Demux1/1 -> Terminator1/1
  B/1 -> Demux1/1
  A/1 -> Demux/1

== system Project_SADC/Attitude determination /TRIAD /product vector3/j-component ==
  A : Inport
  B : Inport  Port=2
  Demux : Demux  Outputs=3
  Demux1 : Demux  Outputs=3
  Product : Product
  Product1 : Product
  Sum : Sum  Inputs=+-
  Terminator : Terminator
  Terminator1 : Terminator
  Out1 : Outport
  wires:
  B/1 -> Demux1/1
  A/1 -> Demux/1
  Demux/3 -> Product/1  "a3"
  Demux1/1 -> Product/2  "b1"
  Demux/1 -> Product1/1  "a1"
  Demux1/3 -> Product1/2  "b3"
  Demux1/2 -> Terminator/1
  Demux/2 -> Terminator1/1
  Product/1 -> Sum/1
  Product1/1 -> Sum/2
  Sum/1 -> Out1/1

== system Project_SADC/Attitude determination /TRIAD /product vector3/k-component1 ==
  A : Inport
  B : Inport  Port=2
  Demux : Demux  Outputs=3
  Demux1 : Demux  Outputs=3
  Product : Product
  Product1 : Product
  Sum : Sum  Inputs=+-
  Terminator : Terminator
  Terminator1 : Terminator
  Out1 : Outport
  wires:
  Sum/1 -> Out1/1
  Product1/1 -> Sum/2
  Product/1 -> Sum/1
  Demux1/2 -> Product/2  "b2"
  A/1 -> Demux/1
  B/1 -> Demux1/1
  Demux/1 -> Product/1  "a1"
  Demux/2 -> Product1/1  "a2"
  Demux1/1 -> Product1/2  "b1"
  Demux1/3 -> Terminator/1  "b3"
  Demux/3 -> Terminator1/1  "a3"

== system Project_SADC/Attitude determination /TRIAD /product vector4/i-component ==
  A : Inport
  B : Inport  Port=2
  Demux : Demux  Outputs=3
  Demux1 : Demux  Outputs=3
  Product : Product
  Product1 : Product
  Sum : Sum  Inputs=+-
  Terminator : Terminator
  Terminator1 : Terminator
  Out2 : Outport
  wires:
  Sum/1 -> Out2/1
  Product1/1 -> Sum/2  "a3b2"
  Demux1/2 -> Product1/2  "b2"
  Product/1 -> Sum/1  "a2b3"
  Demux/2 -> Product/1  "a2"
  Demux/3 -> Product1/1  "a3"
  Demux1/3 -> Product/2  "b3"
  Demux/1 -> Terminator/1  "a1"
  Demux1/1 -> Terminator1/1
  B/1 -> Demux1/1
  A/1 -> Demux/1

== system Project_SADC/Attitude determination /TRIAD /product vector4/j-component ==
  A : Inport
  B : Inport  Port=2
  Demux : Demux  Outputs=3
  Demux1 : Demux  Outputs=3
  Product : Product
  Product1 : Product
  Sum : Sum  Inputs=+-
  Terminator : Terminator
  Terminator1 : Terminator
  Out1 : Outport
  wires:
  B/1 -> Demux1/1
  A/1 -> Demux/1
  Demux/3 -> Product/1  "a3"
  Demux1/1 -> Product/2  "b1"
  Demux/1 -> Product1/1  "a1"
  Demux1/3 -> Product1/2  "b3"
  Demux1/2 -> Terminator/1
  Demux/2 -> Terminator1/1
  Product/1 -> Sum/1
  Product1/1 -> Sum/2
  Sum/1 -> Out1/1

== system Project_SADC/Attitude determination /TRIAD /product vector4/k-component1 ==
  A : Inport
  B : Inport  Port=2
  Demux : Demux  Outputs=3
  Demux1 : Demux  Outputs=3
  Product : Product
  Product1 : Product
  Sum : Sum  Inputs=+-
  Terminator : Terminator
  Terminator1 : Terminator
  Out1 : Outport
  wires:
  Sum/1 -> Out1/1
  Product1/1 -> Sum/2
  Product/1 -> Sum/1
  Demux1/2 -> Product/2  "b2"
  A/1 -> Demux/1
  B/1 -> Demux1/1
  Demux/1 -> Product/1  "a1"
  Demux/2 -> Product1/1  "a2"
  Demux1/1 -> Product1/2  "b1"
  Demux1/3 -> Terminator/1  "b3"
  Demux/3 -> Terminator1/1  "a3"

== system Project_SADC/Attitude determination /TRIAD /product vector5/i-component ==
  A : Inport
  B : Inport  Port=2
  Demux : Demux  Outputs=3
  Demux1 : Demux  Outputs=3
  Product : Product
  Product1 : Product
  Sum : Sum  Inputs=+-
  Terminator : Terminator
  Terminator1 : Terminator
  Out2 : Outport
  wires:
  A/1 -> Demux/1
  B/1 -> Demux1/1
  Demux1/1 -> Terminator1/1
  Demux/1 -> Terminator/1  "a1"
  Demux1/3 -> Product/2  "b3"
  Demux/3 -> Product1/1  "a3"
  Demux/2 -> Product/1  "a2"
  Product/1 -> Sum/1  "a2b3"
  Demux1/2 -> Product1/2  "b2"
  Product1/1 -> Sum/2  "a3b2"
  Sum/1 -> Out2/1

== system Project_SADC/Attitude determination /TRIAD /product vector5/j-component ==
  A : Inport
  B : Inport  Port=2
  Demux : Demux  Outputs=3
  Demux1 : Demux  Outputs=3
  Product : Product
  Product1 : Product
  Sum : Sum  Inputs=+-
  Terminator : Terminator
  Terminator1 : Terminator
  Out1 : Outport
  wires:
  Sum/1 -> Out1/1
  Product1/1 -> Sum/2
  Product/1 -> Sum/1
  Demux/2 -> Terminator1/1
  Demux1/2 -> Terminator/1
  Demux1/3 -> Product1/2  "b3"
  Demux/1 -> Product1/1  "a1"
  Demux1/1 -> Product/2  "b1"
  Demux/3 -> Product/1  "a3"
  A/1 -> Demux/1
  B/1 -> Demux1/1

== system Project_SADC/Attitude determination /TRIAD /product vector5/k-component1 ==
  A : Inport
  B : Inport  Port=2
  Demux : Demux  Outputs=3
  Demux1 : Demux  Outputs=3
  Product : Product
  Product1 : Product
  Sum : Sum  Inputs=+-
  Terminator : Terminator
  Terminator1 : Terminator
  Out1 : Outport
  wires:
  Demux/3 -> Terminator1/1  "a3"
  Demux1/3 -> Terminator/1  "b3"
  Demux1/1 -> Product1/2  "b1"
  Demux/2 -> Product1/1  "a2"
  Demux/1 -> Product/1  "a1"
  B/1 -> Demux1/1
  A/1 -> Demux/1
  Demux1/2 -> Product/2  "b2"
  Product/1 -> Sum/1
  Product1/1 -> Sum/2
  Sum/1 -> Out1/1

== system Project_SADC/Attitude determination /selection sensor/Vector norm3/norm_vector ==
  u : Inport
  Demux : Demux  Outputs=3
  Square : Math  Operator=square  SaturateOnIntegerOverflow=on
  Square Root : Sqrt  SaturateOnIntegerOverflow=on
  Square1 : Math  Operator=square  SaturateOnIntegerOverflow=on
  Square3 : Math  Operator=square  SaturateOnIntegerOverflow=on
  Sum : Sum  Inputs=+++
  |u| : Outport
  wires:
  Square Root/1 -> |u|/1
  Sum/1 -> Square Root/1
  Square1/1 -> Sum/2
  Square3/1 -> Sum/3
  Square/1 -> Sum/1
  Demux/3 -> Square3/1
  Demux/2 -> Square1/1
  Demux/1 -> Square/1
  u/1 -> Demux/1

== system Project_SADC/External torques/GG torque/Vector norm/norm_vector ==
  u : Inport
  Demux : Demux  Outputs=3
  Square : Math  Operator=square  SaturateOnIntegerOverflow=on
  Square Root : Sqrt  SaturateOnIntegerOverflow=on
  Square1 : Math  Operator=square  SaturateOnIntegerOverflow=on
  Square3 : Math  Operator=square  SaturateOnIntegerOverflow=on
  Sum : Sum  Inputs=+++
  |u| : Outport
  wires:
  u/1 -> Demux/1
  Demux/1 -> Square/1
  Demux/2 -> Square1/1
  Demux/3 -> Square3/1
  Square/1 -> Sum/1
  Square3/1 -> Sum/3
  Square1/1 -> Sum/2
  Sum/1 -> Square Root/1
  Square Root/1 -> |u|/1

== system Project_SADC/External torques/GG torque/product vector/i-component ==
  A : Inport
  B : Inport  Port=2
  Demux : Demux  Outputs=3
  Demux1 : Demux  Outputs=3
  Product : Product
  Product1 : Product
  Sum : Sum  Inputs=+-
  Terminator : Terminator
  Terminator1 : Terminator
  Out2 : Outport
  wires:
  Sum/1 -> Out2/1
  Product1/1 -> Sum/2  "a3b2"
  Demux1/2 -> Product1/2  "b2"
  Product/1 -> Sum/1  "a2b3"
  Demux/2 -> Product/1  "a2"
  Demux/3 -> Product1/1  "a3"
  Demux1/3 -> Product/2  "b3"
  Demux/1 -> Terminator/1  "a1"
  Demux1/1 -> Terminator1/1
  B/1 -> Demux1/1
  A/1 -> Demux/1

== system Project_SADC/External torques/GG torque/product vector/j-component ==
  A : Inport
  B : Inport  Port=2
  Demux : Demux  Outputs=3
  Demux1 : Demux  Outputs=3
  Product : Product
  Product1 : Product
  Sum : Sum  Inputs=+-
  Terminator : Terminator
  Terminator1 : Terminator
  Out1 : Outport
  wires:
  B/1 -> Demux1/1
  A/1 -> Demux/1
  Demux/3 -> Product/1  "a3"
  Demux1/1 -> Product/2  "b1"
  Demux/1 -> Product1/1  "a1"
  Demux1/3 -> Product1/2  "b3"
  Demux1/2 -> Terminator/1
  Demux/2 -> Terminator1/1
  Product/1 -> Sum/1
  Product1/1 -> Sum/2
  Sum/1 -> Out1/1

== system Project_SADC/External torques/GG torque/product vector/k-component1 ==
  A : Inport
  B : Inport  Port=2
  Demux : Demux  Outputs=3
  Demux1 : Demux  Outputs=3
  Product : Product
  Product1 : Product
  Sum : Sum  Inputs=+-
  Terminator : Terminator
  Terminator1 : Terminator
  Out1 : Outport
  wires:
  Sum/1 -> Out1/1
  Product1/1 -> Sum/2
  Product/1 -> Sum/1
  Demux1/2 -> Product/2  "b2"
  A/1 -> Demux/1
  B/1 -> Demux1/1
  Demux/1 -> Product/1  "a1"
  Demux/2 -> Product1/1  "a2"
  Demux1/1 -> Product1/2  "b1"
  Demux1/3 -> Terminator/1  "b3"
  Demux/3 -> Terminator1/1  "a3"

== system Project_SADC/External torques/Magnetic torque/mag_field in inertial/Vector norm1 ==
  u : Inport
  Divide : Product  Inputs=*/
  norm_vector : Subsystem
  u_versor : Outport
  ||u|| : Outport  Port=2
  wires:
  u/1 -> Divide/1, norm_vector/1(u)
  norm_vector/1(|u|) -> ||u||/1, Divide/2
  Divide/1 -> u_versor/1

== system Project_SADC/External torques/Magnetic torque/mag_field in inertial/m_versor ==
  time : Inport
  Constant : Constant  Value=data.we
  Constant1 : Constant  Value=11.5
  Cos : Trigonometry  Operator=cos
  Cos1 : Trigonometry  Operator=cos
  Degrees to Radians : simulink_extras/Transformations/Degrees to Radians
  Mux : Mux  Inputs=3
  Product : Product
  Product1 : Product
  Product2 : Product
  Reshape : Reshape  OutputDimensionality=Column vector (2-D)
  Sin : Trigonometry
  Sin1 : Trigonometry
  m : Outport
  wires:
  Constant1/1 -> Degrees to Radians/1
  Constant/1 -> Product/2
  time/1 -> Product/1
  Product/1 -> Sin1/1, Cos1/1
  Cos1/1 -> Product1/2
  Degrees to Radians/1 -> Cos/1, Sin/1
  Sin/1 -> Product2/1, Product1/1
  Sin1/1 -> Product2/2
  Product2/1 -> Mux/2
  Cos/1 -> Mux/3
  Product1/1 -> Mux/1
  Mux/1 -> Reshape/1
  Reshape/1 -> m/1

== system Project_SADC/External torques/Magnetic torque/product vector2/i-component ==
  A : Inport
  B : Inport  Port=2
  Demux : Demux  Outputs=3
  Demux1 : Demux  Outputs=3
  Product : Product
  Product1 : Product
  Sum : Sum  Inputs=+-
  Terminator : Terminator
  Terminator1 : Terminator
  Out2 : Outport
  wires:
  A/1 -> Demux/1
  B/1 -> Demux1/1
  Demux1/1 -> Terminator1/1
  Demux/1 -> Terminator/1  "a1"
  Demux1/3 -> Product/2  "b3"
  Demux/3 -> Product1/1  "a3"
  Demux/2 -> Product/1  "a2"
  Product/1 -> Sum/1  "a2b3"
  Demux1/2 -> Product1/2  "b2"
  Product1/1 -> Sum/2  "a3b2"
  Sum/1 -> Out2/1

== system Project_SADC/External torques/Magnetic torque/product vector2/j-component ==
  A : Inport
  B : Inport  Port=2
  Demux : Demux  Outputs=3
  Demux1 : Demux  Outputs=3
  Product : Product
  Product1 : Product
  Sum : Sum  Inputs=+-
  Terminator : Terminator
  Terminator1 : Terminator
  Out1 : Outport
  wires:
  Sum/1 -> Out1/1
  Product1/1 -> Sum/2
  Product/1 -> Sum/1
  Demux/2 -> Terminator1/1
  Demux1/2 -> Terminator/1
  Demux1/3 -> Product1/2  "b3"
  Demux/1 -> Product1/1  "a1"
  Demux1/1 -> Product/2  "b1"
  Demux/3 -> Product/1  "a3"
  A/1 -> Demux/1
  B/1 -> Demux1/1

== system Project_SADC/External torques/Magnetic torque/product vector2/k-component1 ==
  A : Inport
  B : Inport  Port=2
  Demux : Demux  Outputs=3
  Demux1 : Demux  Outputs=3
  Product : Product
  Product1 : Product
  Sum : Sum  Inputs=+-
  Terminator : Terminator
  Terminator1 : Terminator
  Out1 : Outport
  wires:
  Demux/3 -> Terminator1/1  "a3"
  Demux1/3 -> Terminator/1  "b3"
  Demux1/1 -> Product1/2  "b1"
  Demux/2 -> Product1/1  "a2"
  Demux/1 -> Product/1  "a1"
  B/1 -> Demux1/1
  A/1 -> Demux/1
  Demux1/2 -> Product/2  "b2"
  Product/1 -> Sum/1
  Product1/1 -> Sum/2
  Sum/1 -> Out1/1

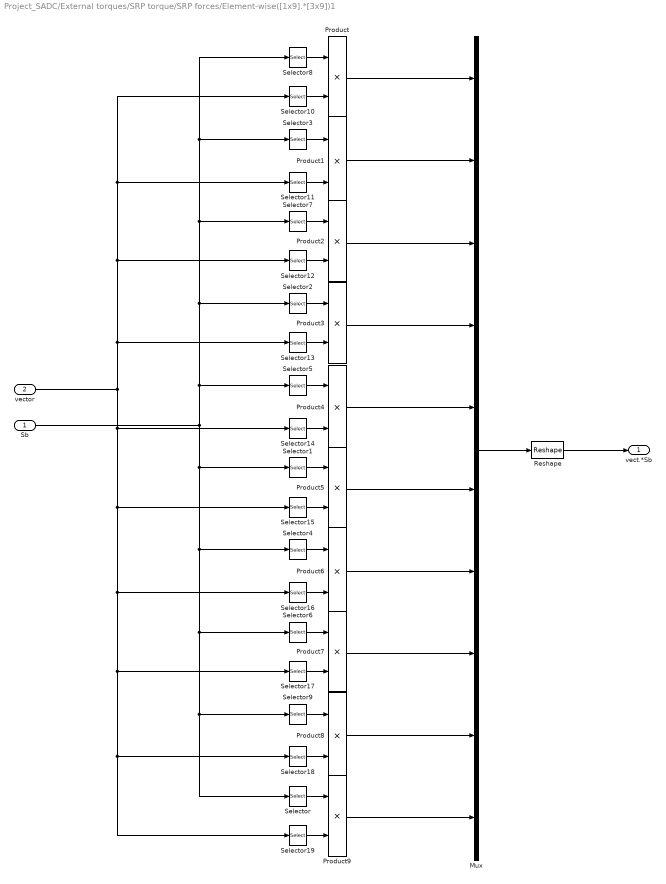
== system Project_SADC/External torques/SRP torque/SRP forces/Element-wise([1x9].*[3x9])1 ==
  Sb : Inport
  vector : Inport  Port=2
  Mux : Mux  Inputs=10
  Product{,1..9} (10 alike) : Product
  Reshape : Reshape  OutputDimensionality=Customize  OutputDimensions=[3,10]
  Selector : Selector  NumberOfDimensions=2  InputPortWidth=3  IndexOptions=Index vector (dialog),Index vector (dialog)  Indices=[1 2 3],10  OutputSizes=1,1
  Selector1 : Selector  NumberOfDimensions=2  InputPortWidth=3  IndexOptions=Index vector (dialog),Index vector (dialog)  Indices=[1 2 3],6  OutputSizes=1,1
  Selector10 : Selector  InputPortWidth=10  IndexOptions=Index vector (dialog)  Indices=1  OutputSizes=1
  Selector11 : Selector  InputPortWidth=10  IndexOptions=Index vector (dialog)  Indices=2  OutputSizes=1
  Selector12 : Selector  InputPortWidth=10  IndexOptions=Index vector (dialog)  Indices=3  OutputSizes=1
  Selector13 : Selector  InputPortWidth=10  IndexOptions=Index vector (dialog)  Indices=4  OutputSizes=1
  Selector14 : Selector  InputPortWidth=10  IndexOptions=Index vector (dialog)  Indices=5  OutputSizes=1
  Selector15 : Selector  InputPortWidth=10  IndexOptions=Index vector (dialog)  Indices=6  OutputSizes=1
  Selector16 : Selector  InputPortWidth=10  IndexOptions=Index vector (dialog)  Indices=7  OutputSizes=1
  Selector17 : Selector  InputPortWidth=10  IndexOptions=Index vector (dialog)  Indices=8  OutputSizes=1
  Selector18 : Selector  InputPortWidth=10  IndexOptions=Index vector (dialog)  Indices=9  OutputSizes=1
  Selector19 : Selector  InputPortWidth=10  IndexOptions=Index vector (dialog)  Indices=10  OutputSizes=1
  Selector2 : Selector  NumberOfDimensions=2  InputPortWidth=3  IndexOptions=Index vector (dialog),Index vector (dialog)  Indices=[1 2 3],4  OutputSizes=1,1
  Selector3 : Selector  NumberOfDimensions=2  InputPortWidth=3  IndexOptions=Index vector (dialog),Index vector (dialog)  Indices=[1 2 3],2  OutputSizes=1,1
  Selector4 : Selector  NumberOfDimensions=2  InputPortWidth=3  IndexOptions=Index vector (dialog),Index vector (dialog)  Indices=[1 2 3],7  OutputSizes=1,1
  Selector5 : Selector  NumberOfDimensions=2  InputPortWidth=3  IndexOptions=Index vector (dialog),Index vector (dialog)  Indices=[1 2 3],5  OutputSizes=1,1
  Selector6 : Selector  NumberOfDimensions=2  InputPortWidth=3  IndexOptions=Index vector (dialog),Index vector (dialog)  Indices=[1 2 3],8  OutputSizes=1,1
  Selector7 : Selector  NumberOfDimensions=2  InputPortWidth=3  IndexOptions=Index vector (dialog),Index vector (dialog)  Indices=[1 2 3],3  OutputSizes=1,1
  Selector8 : Selector  NumberOfDimensions=2  InputPortWidth=3  IndexOptions=Index vector (dialog),Index vector (dialog)  Indices=[1 2 3],1  OutputSizes=1,1
  Selector9 : Selector  NumberOfDimensions=2  InputPortWidth=3  IndexOptions=Index vector (dialog),Index vector (dialog)  Indices=[1 2 3],9  OutputSizes=1,1
  vect.*Sb : Outport
  wires:
  Product/1 -> Mux/1
  Product1/1 -> Mux/2
  Product2/1 -> Mux/3
  Product3/1 -> Mux/4
  Product4/1 -> Mux/5
  Product6/1 -> Mux/7
  Product5/1 -> Mux/6
  Product7/1 -> Mux/8
  Product8/1 -> Mux/9
  Product9/1 -> Mux/10
  Selector3/1 -> Product1/1
  Selector11/1 -> Product1/2
  Selector7/1 -> Product2/1
  Selector12/1 -> Product2/2
  Selector2/1 -> Product3/1
  Selector13/1 -> Product3/2
  Selector5/1 -> Product4/1
  Selector14/1 -> Product4/2
  Selector1/1 -> Product5/1
  Selector15/1 -> Product5/2
  Selector4/1 -> Product6/1
  Selector16/1 -> Product6/2
  Selector6/1 -> Product7/1
  Selector17/1 -> Product7/2
  Selector18/1 -> Product8/2
  Selector9/1 -> Product8/1
  Selector19/1 -> Product9/2
  Selector/1 -> Product9/1
  Selector10/1 -> Product/2
  Selector8/1 -> Product/1
  vector/1 -> Selector10/1, Selector11/1, Selector12/1, Selector13/1, Selector14/1, Selector15/1, Selector16/1, Selector17/1, Selector18/1, Selector19/1
  Sb/1 -> Selector9/1, Selector/1, Selector6/1, Selector4/1, Selector1/1, Selector8/1, Selector3/1, Selector7/1, Selector2/1, Selector5/1
  Reshape/1 -> vect.*Sb/1
  Mux/1 -> Reshape/1
